simulink model "HW2_Q1"  (R2023a)
settings: Solver=VariableStepAuto  StartTime=0.0  StopTime=10.0  RelTol=1e-3
model workspace (MAT data in the model file):
  K = 1
  M = 2
  b = 1
  k = 1
  m = 1
settings Model: Creator=kaleb  LastModifiedBy=kaleb

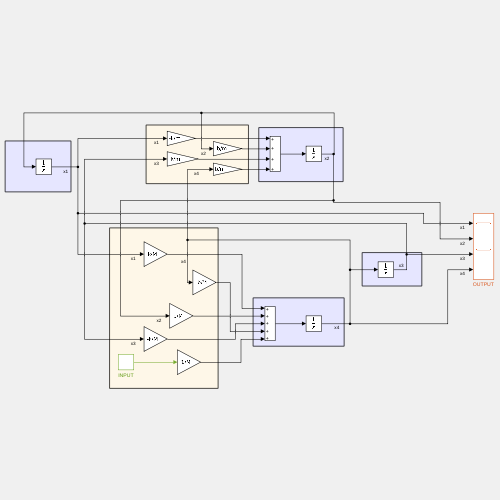
[thumbnail: Simulink's stored preview of the top-level diagram]
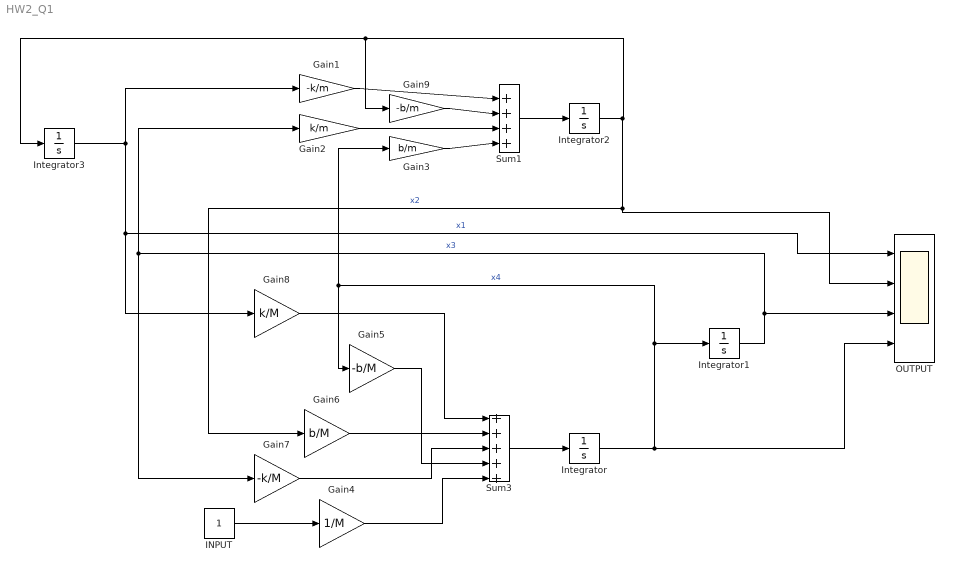
== system HW2_Q1 ==
  Gain1 : Gain  Gain=-k/m
  Gain2 : Gain  Gain=k/m
  Gain3 : Gain  Gain=b/m
  Gain4 : Gain  Gain=1/M
  Gain5 : Gain  Gain=-b/M
  Gain6 : Gain  Gain=b/M
  Gain7 : Gain  Gain=-k/M
  Gain8 : Gain  Gain=k/M
  Gain9 : Gain  Gain=-b/m
  INPUT : Constant
  Integrator{,1..3} (4 alike) : Integrator
  OUTPUT : Scope  NumInputPorts=4
  Sum1 : Sum  Inputs=+|+|+|+
  Sum3 : Sum  Inputs=+++++
  wires:
  Integrator/1 -> OUTPUT/4, Integrator1/1, Gain3/1, Gain5/1  "x4"
  Sum3/1 -> Integrator/1
  Integrator1/1 -> OUTPUT/3, Gain2/1, Gain7/1  "x3"
  Gain7/1 -> Sum3/3
  Gain6/1 -> Sum3/2
  Gain8/1 -> Sum3/1
  Gain5/1 -> Sum3/4
  INPUT/1 -> Gain4/1
  Sum1/1 -> Integrator2/1
  Gain9/1 -> Sum1/2
  Integrator3/1 -> Gain8/1, OUTPUT/1, Gain1/1  "x1"
  Gain1/1 -> Sum1/1
  Gain2/1 -> Sum1/3
  Gain3/1 -> Sum1/4
  Integrator2/1 -> OUTPUT/2, Gain6/1, Integrator3/1, Gain9/1  "x2"
  Gain4/1 -> Sum3/5
